simulink model "switchDown"  (Simulink 7.4)
settings: Solver=ode45  StartTime=0.0  StopTime=10.0  RelTol=1e-3
settings Model: Creator=wangwig  LastModifiedBy=wangwig

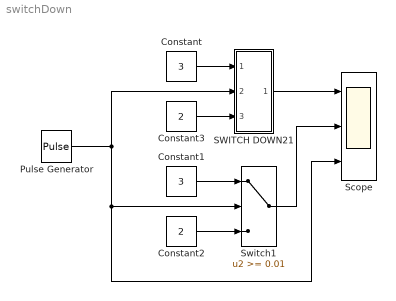
== system switchDown ==
  Constant : Constant  Value=3  OutDataType=fixdt(1, 16)  OutScaling=2^0
  Constant1 : Constant  Value=3  OutDataType=fixdt(1, 16)  OutScaling=2^0
  Constant2 : Constant  Value=2  OutDataType=fixdt(1, 16)  OutScaling=2^0
  Constant3 : Constant  Value=2  OutDataType=fixdt(1, 16)  OutScaling=2^0
  Pulse Generator : DiscretePulseGenerator  PulseType=Time based  Amplitude=1  Period=1  PulseWidth=33  PhaseDelay=0  SampleTime=1
  SWITCH DOWN21 : Subsystem
      mask Type: SwitchDown
      mask Description: Output is input 1 when control input is set to 0; otherwise if control input is set to 1 output is input 2.
      mask Display:
      | plot([0 0.2],[0.5 0.5]);
      | plot([0 0.4],[0.75 0.75])
      | plot([0 0.4],[0.25 0.25])
      | plot([0.8 1],[0.5 0.5])
      | plot([0.2 0.2],[0.4 0.6])
      | plot([0.4 0.4 0.46 0.46 0.4],[0.78 0.72 0.72 0.78 0.78])
      | plot([0.4 0.4 0.46 0.46 0.4],[0.28 0.22 0.22 0.28 0.28])
      | plot([0.46 0.8],[0.75 0.5])
      | plot([0.63 0.63],[0.85 0.13])
      | plot([0.60 0.635 0.68],[0.19 0.13 0.19])
  Scope : Scope  NumInputPorts=3
      settings: YMin=-5~-5~-5  YMax=5~5~5
  Switch1 : Switch  Threshold=0.01  OutDataType=fixdt(1, 16)  OutScaling=2^0
  wires:
  SWITCH DOWN21/1(Out) -> Scope/1
  Switch1/1 -> Scope/2
  Constant/1 -> SWITCH DOWN21/1(In1)
  Constant1/1 -> Switch1/1
  Constant2/1 -> Switch1/3
  Constant3/1 -> SWITCH DOWN21/3(In2)
  Pulse Generator/1 -> SWITCH DOWN21/2(CtrlIn), Scope/3, Switch1/2

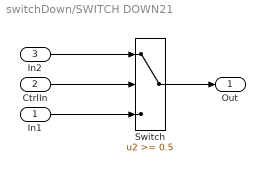
== system switchDown/SWITCH DOWN21 ==
  In1 : Inport  OutDataType=sfix(16)  OutScaling=2^0
  CtrlIn : Inport  Port=2  OutDataType=sfix(16)  OutScaling=2^0
  In2 : Inport  Port=3  OutDataType=sfix(16)  OutScaling=2^0
  Switch : Switch  Threshold=0.5  OutDataType=fixdt(1, 16)  OutScaling=2^0  mask(TL_Switch){data=struct('comment',struct('text','','placement',1),'logdata',struct('maxnumvals',inf,'plotchannels',[],'loggingmode',3,'channels',1),'output',struct('width',1,'name','$S_$B','unit','','type','Int16','offset',0,'max',NaN,'min',NaN,'freeze',1,'lsb',2^-4,'arb',0,'class','default','address','','description','','autoscalingmode',1,'lowerheadroom',1,'upperheadroom',1,'headroomunit','bit','checkmin',0,'checkmax',0,'show',0,'variable','','scaling','','keepdatatype',1,'castoutput',0),'threshold',struct('width',1,'name','$S_$B_threshold','unit','','type','Int16','offset',0,'max',NaN,'min',NaN,'freeze',1,'lsb',1,'arb',0,'class','default','address','','description','','value','0.5','scalar',0,'variable','','scaling','','keepdatatype',1,'criteria',1),'date',733278.36129861115,'scalingvalid',0)}
      settings: CopyFcn=if exist('tl_reset_reviewflag') == 2, tl_reset_reviewflag(gcbh); end  DeleteFcn=if exist('delete_tlblock','file')==2,delete_tlblock(gcbh);end  NameChangeFcn=if exist('rename_tlblock','file')==2,rename_tlblock(gcbh);end  OpenFcn=if exist('tl_open_blockdlg','file')==2,tl_open_blockdlg(gcbh);else,open_system(gcbh,'parameter');end
      mask Help: eval(['if exist(''tl_online_help'',''file'') == 2, tl_online_help(''Topic'',''TL_Switch''),else, web([''jar:file:///'',matlabroot,''/help/toolbox/simulink/help.jar!/slref/' lower(get_param(gcbh,'Blocktype')) '.html''], ''-helpbrowser''),end'])
      mask Display: plot([-0.05, 1.05, NaN, -0.05, 1.05],[.01, .01, NaN, .99, .99])
  Out : Outport  OutDataType=sfix(16)  OutScaling=2^0
  wires:
  In1/1 -> Switch/3
  In2/1 -> Switch/1
  CtrlIn/1 -> Switch/2
  Switch/1 -> Out/1
